simulink library "ERG_lib"  (R2018b)
settings: Solver=VariableStepAuto  StartTime=0.0  StopTime=10.0  RelTol=1e-3
undefined symbols (not defined in the file or in its folder): x0
libraries: $bdroot x2
settings Model: Creator=Admin  LastModifiedBy=Admin
settings SFSimCC: SimUseLocalCustomCode=off
settings RTWCC: RTWUseLocalCustomCode=off
settings CodeAppCC: StateflowObjectComments=on

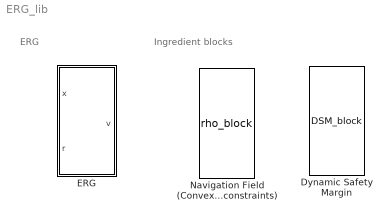
== system ERG_lib ==
  note: ERG
  note: Ingredient blocks
  Dynamic Safety Margin : M-S-Function  FunctionName=DSM_block  Parameters=erg_param  mask(Dynamic Safety Margin){erg_param=[]}
      mask prompts: erg_param "ERGController object:"
      mask help: This block computes the Dynamic Safety Margin for a LTI system subject to linear constraints controlled with an ERG.
      mask Display:
      | port_label('input',1,'x')
      | port_label('input',2,'v')
      | port_label('output',1,'delta')
  ERG : Subsystem  mask(ERG){erg_param=[], kappa_param=1000}
      mask prompts: erg_param "ERGController object:"; kappa_param "Gain (kappa):"
      mask help: This block is an Explicit Reference Governor for an LTI system subject to linear constraints.
      mask Display:
      | port_label('input',1,'x')
      | port_label('input',2,'r')
      | port_label('output',1,'v')
  Navigation Field (Convex constraints) : M-S-Function  FunctionName=rho_block  Parameters=erg_param  mask(Navigation Field (Convex constraints)){erg_param=[]}
      mask prompts: erg_param "ERGController object"
      mask help: This block computes the Navigation Field for a LTI system subject to linear constraints controlled with an ERG.
      mask Display:
      | port_label('input',1,'r')
      | port_label('input',2,'v')
      | port_label('input',3,'x')
      | port_label('output',1,'rho')

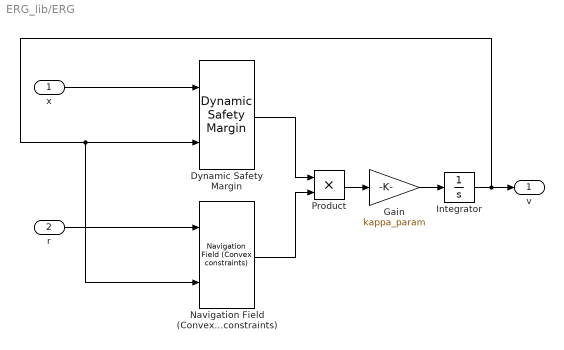
== system ERG_lib/ERG ==
  x : Inport
  r : Inport  Port=2
  Dynamic Safety Margin : $bdroot/Dynamic Safety Margin  erg_param=erg_param
  Gain : Gain  Gain=kappa_param
  Integrator : Integrator  InitialCondition=erg_param.C*x0
  Navigation Field (Convex constraints) : $bdroot/Navigation Field (Convex constraints)  erg_param=erg_param
  Product : Product
  v : Outport
  wires:
  r/1 -> Navigation Field (Convex constraints)/1
  Integrator/1 -> v/1, Navigation Field (Convex constraints)/2, Dynamic Safety Margin/2
  x/1 -> Dynamic Safety Margin/1
  Navigation Field (Convex constraints)/1 -> Product/2
  Dynamic Safety Margin/1 -> Product/1
  Gain/1 -> Integrator/1
  Product/1 -> Gain/1
